simulink model "BLOC_FA_TQ_to_F_BRAKE"  (R2016a)
settings: Solver=VariableStepAuto  StartTime=0.0  StopTime=10.0  RelTol=1e-3
undefined symbols (not defined in the file): pla_wheel_radius
settings Model: Creator=Florent  LastModifiedBy=Florent
settings OptimizationCC: DefaultParameterBehavior=Inlined  OptimizeModelRefInitCode=on  LifeSpan=1
settings RTWCC: SystemTargetFile=ert.tlc  TemplateMakefile=ert_default_tmf  GenerateReport=on  IncludeHyperlinkInReport=on  LaunchReport=on  TargetLang=C++  GenerateTraceInfo=on  GenerateTraceReport=on  GenerateTraceReportSl=on  GenerateTraceReportSf=on  GenerateTraceReportEml=on
settings CodeAppCC: ForceParamTrailComments=on  OperatorAnnotations=on  SimulinkDataObjDesc=on  SFDataObjDesc=on  MATLABFcnDesc=on  InsertBlockDesc=on  MATLABSourceComments=on
settings ERTTargetCC: GenerateSampleERTMain=on  MultiInstanceERTCode=on  CodeInterfacePackaging=C++ class  InlinedParameterPlacement=NonHierarchical  RootIOFormat=Structure reference  ERTCustomFileTemplate=example_file_process.tlc

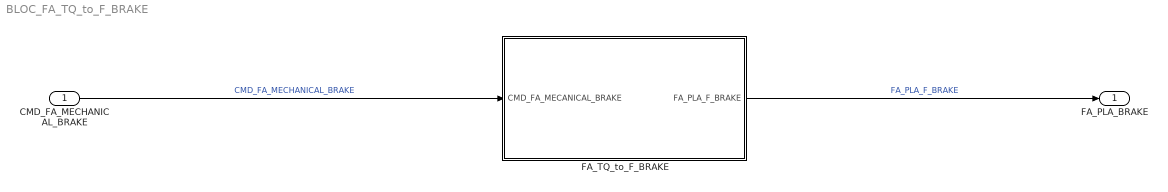
== system BLOC_FA_TQ_to_F_BRAKE ==
  CMD_FA_MECHANICAL_BRAKE : Inport
  FA_TQ_to_F_BRAKE : Subsystem  TreatAsAtomicUnit=on
  FA_PLA_BRAKE : Outport
  wires:
  CMD_FA_MECHANICAL_BRAKE/1 -> FA_TQ_to_F_BRAKE/1(CMD_FA_MECANICAL_BRAKE)  "CMD_FA_MECHANICAL_BRAKE"
  FA_TQ_to_F_BRAKE/1(FA_PLA_F_BRAKE) -> FA_PLA_BRAKE/1  "FA_PLA_F_BRAKE"

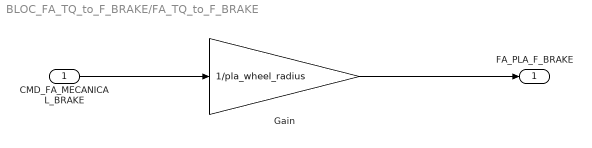
== system BLOC_FA_TQ_to_F_BRAKE/FA_TQ_to_F_BRAKE ==
  CMD_FA_MECANICAL_BRAKE : Inport
  Gain : Gain  Gain=1/pla_wheel_radius
  FA_PLA_F_BRAKE : Outport
  wires:
  CMD_FA_MECANICAL_BRAKE/1 -> Gain/1
  Gain/1 -> FA_PLA_F_BRAKE/1
